simulink model "motordrv_currentsen"  (R2018b)
settings: Solver=VariableStepAuto  StartTime=0.0  StopTime=Endtime  RelTol=1e-3
values from neighbouring files (symbols this model uses):
  alpha_i = 5/37.5    (= 0.133333333333)    [drv_sen_sim.m]    (also in plant_model_sim.m)
  i_M_d = 3    [drv_sen_sim.m]    (also in plant_model_sim.m)
  u_M_d = 10    [drv_sen_sim.m]    (also in plant_model_sim.m)
  Vin = 24    [drv_sen_sim.m]    (also in plant_model_sim.m)
libraries: simulink x2
settings Model: Creator=nharada  LastModifiedBy=nharada

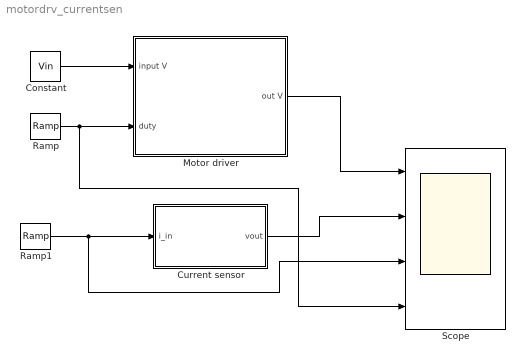
== system motordrv_currentsen ==
  Constant : Constant  Value=Vin
  Current sensor : Subsystem
  Motor driver : Subsystem
  Ramp : simulink/Sources/Ramp  slope=u_M_d  start=0  InitialOutput=0
  Ramp1 : simulink/Sources/Ramp  slope=i_M_d  start=0  InitialOutput=0
  Scope : Scope  NumInputPorts=4
  wires:
  Constant/1 -> Motor driver/1(input V)
  Ramp/1 -> Scope/4, Motor driver/2(duty)
  Ramp1/1 -> Scope/3, Current sensor/1(i_in)
  Motor driver/1(out V) -> Scope/1
  Current sensor/1(vout) -> Scope/2

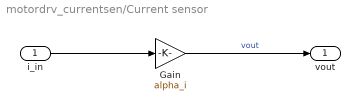
== system motordrv_currentsen/Current sensor ==
  i_in : Inport
  Gain : Gain  Gain=alpha_i
  vout : Outport
  wires:
  Gain/1 -> vout/1  "vout"
  i_in/1 -> Gain/1

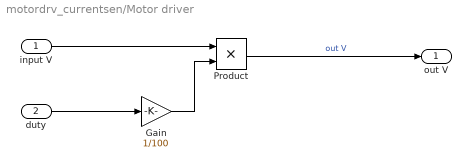
== system motordrv_currentsen/Motor driver ==
  input V : Inport
  duty : Inport  Port=2
  Gain : Gain  Gain=1/100
  Product : Product
  out V : Outport
  wires:
  Gain/1 -> Product/2
  input V/1 -> Product/1
  Product/1 -> out V/1  "out V"
  duty/1 -> Gain/1
